simulink model "RALFJoystick"  (R2018b)
settings: Solver=FixedStepAuto  StartTime=0.0  StopTime=inf  FixedStep=0.05  RelTol=1e-3
model workspace (MAT data in the model file):
  SL_ROS_VariableLengthArrays_MaxSizes.CommonInfo.ArrayTruncateAction = 'EmitWarning'
  SL_ROS_VariableLengthArrays_MaxSizes.MsgTypeMap = containers.Map
  SL_ROS_VariableLengthArrays_MaxSizes.MsgTypeMap.serialization.keys = {'sensor_msgs/Joy'}
  SL_ROS_VariableLengthArrays_MaxSizes.MsgTypeMap.serialization.values{1}(1).PropertyName = 'Axes'
  SL_ROS_VariableLengthArrays_MaxSizes.MsgTypeMap.serialization.values{1}(1).DataType = 'single'
  SL_ROS_VariableLengthArrays_MaxSizes.MsgTypeMap.serialization.values{1}(1).MaxLength = 8
  SL_ROS_VariableLengthArrays_MaxSizes.MsgTypeMap.serialization.values{1}(2).PropertyName = 'Buttons'
  SL_ROS_VariableLengthArrays_MaxSizes.MsgTypeMap.serialization.values{1}(2).DataType = 'int32'
  SL_ROS_VariableLengthArrays_MaxSizes.MsgTypeMap.serialization.values{1}(2).MaxLength = 15
  SL_ROS_VariableLengthArrays_MaxSizes.MsgTypeMap.serialization.uniformity = 0
  SL_ROS_VariableLengthArrays_MaxSizes.MsgTypeMap.serialization.keyType = 'char'
  SL_ROS_VariableLengthArrays_MaxSizes.MsgTypeMap.serialization.valueType = 'any'
undefined symbols (not defined in the file): Axes, Axes_SL_Info, Buttons, Buttons_SL_Info
libraries: robotlib x3, simulink x1
settings Model: Creator=Systemtechnik Labor  LastModifiedBy=Systemtechnik Labor
settings OptimizationCC: EnhancedBackFolding=on  PassReuseOutputArgsAs=Individual arguments  MaxStackSize=64  OptimizeBlockOrder=speed  DifferentSizesBufferReuse=on  OptimizationCustomize=off
settings DebuggingCC: ParameterTunabilityLossMsg=error
settings HardwareCC: ProdBitPerPointer=32  ProdBitPerSizeT=32  ProdBitPerPtrDiffT=32  ProdLargestAtomicFloat=None  ProdIntDivRoundTo=Undefined  ProdEndianess=Unspecified  ProdWordSize=32  ProdHWDeviceType=Generic->Unspecified (assume 32-bit Generic)
settings SFSimCC: MATLABDynamicMemAlloc=off
settings RTWCC: SystemTargetFile=ert.tlc  HardwareBoard=Robot Operating System (ROS)  TLCOptions="-aInlineSetEventsForThisBaseRateFcn=TLC_FALSE -aSuppressMultiTaskScheduler=TLC_FALSE  -aRateBasedStepFcn=0"  TemplateMakefile=ert_default_tmf  GenerateReport=on  Toolchain=Catkin  IncludeHyperlinkInReport=on  LaunchReport=on  TargetLang=C++  GenerateTraceInfo=on  GenerateTraceReport=on  GenerateTraceReportSl=on  GenerateTraceReportSf=on  GenerateTraceReportEml=on
settings CodeAppCC: ForceParamTrailComments=on  IgnoreCustomStorageClasses=off  OperatorAnnotations=on  SimulinkDataObjDesc=on  SFDataObjDesc=on  InsertBlockDesc=on

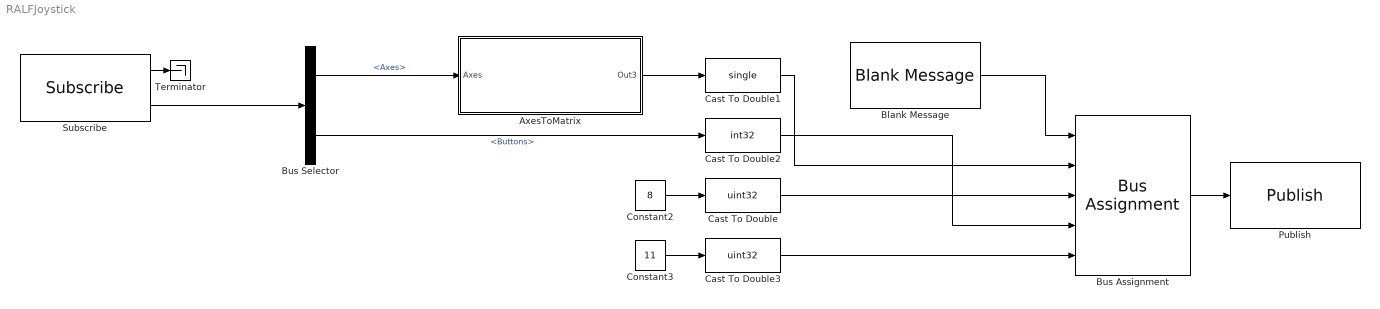
== system RALFJoystick ==
  AxesToMatrix : Subsystem
  Blank Message : robotlib/Blank Message  messageClass=Message  entityType=sensor_msgs/Joy  messageType=sensor_msgs/Joy  SampleTime=inf
      settings: SourceProductBaseCode=RO
  Bus Assignment : BusAssignment  AssignedSignals=Axes,Axes_SL_Info.CurrentLength,Buttons,Buttons_SL_Info.CurrentLength
  Bus Selector : BusSelector  OutputSignals=Axes,Buttons
  Cast To Double : DataTypeConversion  OutDataTypeStr=uint32
  Cast To Double1 : DataTypeConversion  OutDataTypeStr=single
  Cast To Double2 : DataTypeConversion  OutDataTypeStr=int32
  Cast To Double3 : DataTypeConversion  OutDataTypeStr=uint32
  Constant2 : Constant  Value=8
  Constant3 : Constant  Value=11
  Publish : robotlib/Publish  topicSource=Specify your own  topic=/RALFJoy  messageType=sensor_msgs/Joy  messageQueueLength=1
      settings: SourceProductBaseCode=RO
  Subscribe : robotlib/Subscribe  topicSource=Select from ROS network  topic=/joy  messageType=sensor_msgs/Joy  sampleTime=-1  messageQueueLength=1
      settings: SourceProductBaseCode=RO
  Terminator : Terminator
  wires:
  Bus Selector/2 -> Cast To Double2/1  "<Buttons>"
  Bus Selector/1 -> AxesToMatrix/1(Axes)  "<Axes>"
  Subscribe/2 -> Bus Selector/1
  Subscribe/1 -> Terminator/1
  Blank Message/1 -> Bus Assignment/1
  Bus Assignment/1 -> Publish/1
  Constant2/1 -> Cast To Double/1
  Cast To Double1/1 -> Bus Assignment/2
  Cast To Double2/1 -> Bus Assignment/4
  Constant3/1 -> Cast To Double3/1
  Cast To Double/1 -> Bus Assignment/3
  Cast To Double3/1 -> Bus Assignment/5
  AxesToMatrix/1(Out3) -> Cast To Double1/1

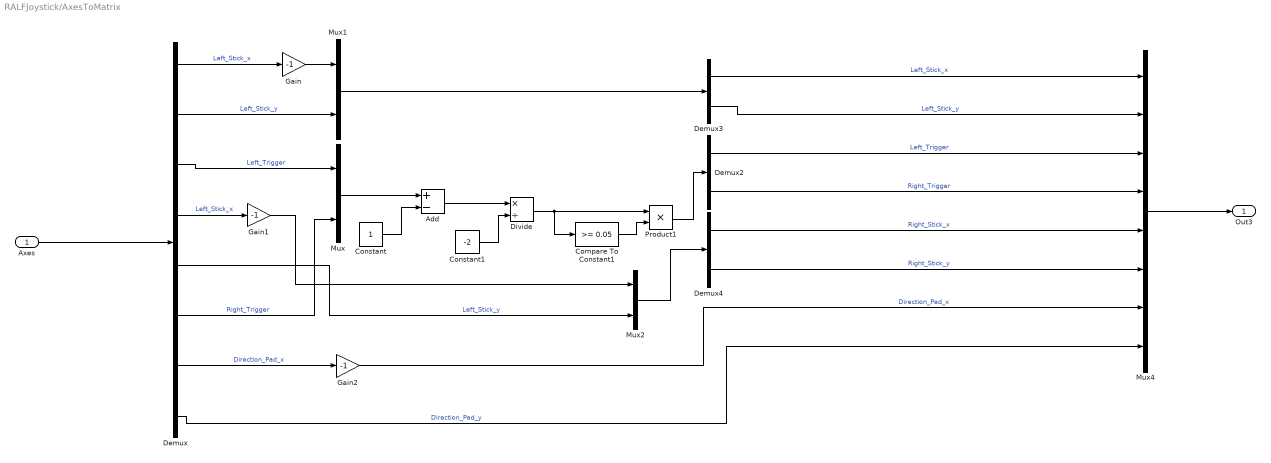
== system RALFJoystick/AxesToMatrix ==
  Axes : Inport
  Add : Sum  Inputs=+-
  Compare To Constant1 : simulink/Logic and Bit Operations/Compare To Constant  relop=>=  const=0.05  OutDataTypeStr=boolean
  Constant : Constant
  Constant1 : Constant  Value=-2
  Demux : Demux  Outputs=8
  Demux2 : Demux  Outputs=2
  Demux3 : Demux  Outputs=2
  Demux4 : Demux  Outputs=2
  Divide : Product  Inputs=*/
  Gain : Gain  Gain=-1
  Gain1 : Gain  Gain=-1
  Gain2 : Gain  Gain=-1
  Mux : Mux  Inputs=2
  Mux1 : Mux  Inputs=2
  Mux2 : Mux  Inputs=2
  Mux4 : Mux  Inputs=8
  Product1 : Product  OutDataTypeStr=single
  Out3 : Outport
  wires:
  Constant1/1 -> Divide/2
  Demux/5 -> Mux2/2  "Left_Stick_y"
  Demux/8 -> Mux4/8  "Direction_Pad_y"
  Mux/1 -> Add/1
  Demux/4 -> Gain1/1  "Left_Stick_x"
  Mux4/1 -> Out3/1
  Demux4/2 -> Mux4/6  "Right_Stick_y"
  Add/1 -> Divide/1
  Gain2/1 -> Mux4/7  "Direction_Pad_x"
  Demux/7 -> Gain2/1  "Direction_Pad_x"
  Demux3/1 -> Mux4/1  "Left_Stick_x"
  Demux/6 -> Mux/2  "Right_Trigger"
  Constant/1 -> Add/2
  Gain/1 -> Mux1/1
  Compare To Constant1/1 -> Product1/2
  Demux2/1 -> Mux4/3  "Left_Trigger"
  Divide/1 -> Compare To Constant1/1, Product1/1
  Product1/1 -> Demux2/1
  Demux3/2 -> Mux4/2  "Left_Stick_y"
  Demux2/2 -> Mux4/4  "Right_Trigger"
  Mux2/1 -> Demux4/1
  Demux4/1 -> Mux4/5  "Right_Stick_x"
  Axes/1 -> Demux/1
  Gain1/1 -> Mux2/1
  Demux/3 -> Mux/1  "Left_Trigger"
  Demux/1 -> Gain/1  "Left_Stick_x"
  Mux1/1 -> Demux3/1
  Demux/2 -> Mux1/2  "Left_Stick_y"
